simulink model "Tire_Force_Observer"  (R2018b)
settings: Solver=FixedStepAuto  StartTime=0.0  StopTime=10.0  RelTol=1e-3
undefined symbols (not defined in the file): A, B, C, DiscIntNeverNeededParam, K, TFO_Ts
settings Model: Creator=univ4123  LastModifiedBy=univ4123
settings RTWCC: GenCodeOnly=on  Toolchain=MinGW64 | gmake (64-bit Windows)

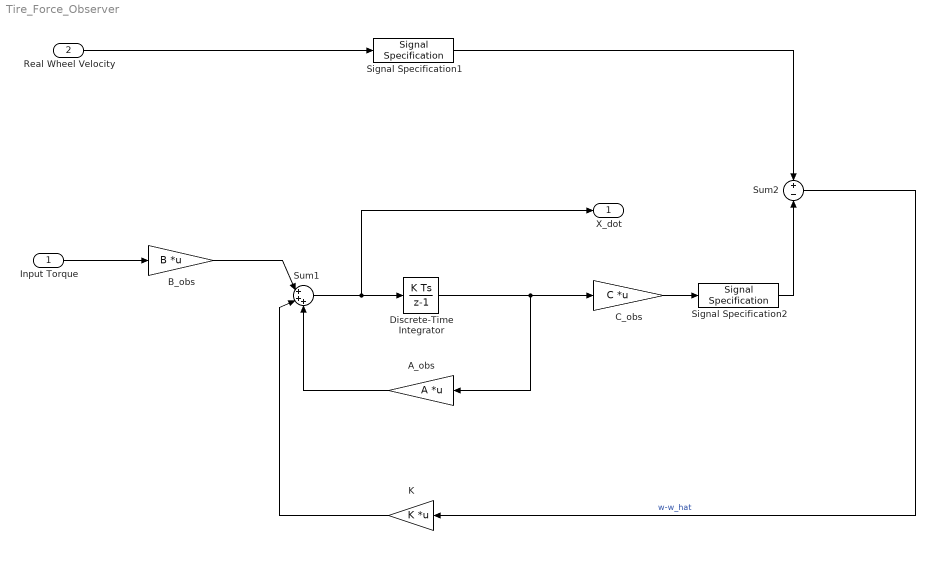
== system Tire_Force_Observer ==
  Input Torque : Inport
  Real Wheel Velocity : Inport  Port=2
  A_obs : Gain  Gain=A  Multiplication=Matrix(K*u) (u vector)
  B_obs : Gain  Gain=B  Multiplication=Matrix(K*u) (u vector)
  C_obs : Gain  Gain=C  Multiplication=Matrix(K*u) (u vector)
  Discrete-Time Integrator : DiscreteIntegrator  SampleTime=TFO_Ts  ICPrevOutput=DiscIntNeverNeededParam  ICPrevScaledInput=DiscIntNeverNeededParam
  K : Gain  Gain=K  Multiplication=Matrix(K*u)
  Signal Specification1 : SignalSpecification  Dimensions=[2 1]
  Signal Specification2 : SignalSpecification  Dimensions=[2 1]
  Sum1 : Sum  Inputs=|+++
  Sum2 : Sum  Inputs=+|-
  X_dot : Outport
  wires:
  Sum1/1 -> X_dot/1, Discrete-Time Integrator/1
  A_obs/1 -> Sum1/3
  K/1 -> Sum1/2
  C_obs/1 -> Signal Specification2/1
  B_obs/1 -> Sum1/1
  Sum2/1 -> K/1  "w-w_hat"
  Discrete-Time Integrator/1 -> A_obs/1, C_obs/1
  Input Torque/1 -> B_obs/1
  Real Wheel Velocity/1 -> Signal Specification1/1
  Signal Specification1/1 -> Sum2/1
  Signal Specification2/1 -> Sum2/2
